simulink model "test_pi_av_formation_event_gazebodirected23a"  (R2023a)
settings: Solver=FixedStepAuto  StartTime=0.0  StopTime=inf  RelTol=1e-3
undefined symbols (not defined in the file or in its folder): angular, DiscIntNeverNeededParam, linear
libraries: ros2lib x28, simulink x8, robotcorelib x8
(part 1 of 4)
settings Model: Creator=johvany  LastModifiedBy=l15
settings OptimizationCC: EnhancedBackFolding=on  PassReuseOutputArgsThreshold=0  ZeroExternalMemoryAtStartup=off  ZeroInternalMemoryAtStartup=off  MaxStackSize=64  OptimizeBlockOrder=speed  DifferentSizesBufferReuse=on  OptimizationCustomize=off
settings DebuggingCC: ParameterTunabilityLossMsg=error
settings HardwareCC: ProdBitPerLong=64  ProdHWDeviceType=Intel->x86-64 (Linux 64)  UseEmbeddedCoderFeatures=off
settings SFSimCC: MATLABDynamicMemAlloc=off
settings RTWCC: Description=Embedded Coder  SystemTargetFile=ert.tlc  HardwareBoard=Robot Operating System 2 (ROS 2)  TLCOptions="-aInlineSetEventsForThisBaseRateFcn=TLC_FALSE -aSuppressMultiTaskScheduler=TLC_FALSE  -aRateBasedStepFcn=0"  TemplateMakefile=ert_default_tmf  Toolchain=Colcon Tools  TargetLang=C++
settings CodeAppCC: ForceParamTrailComments=on  OperatorAnnotations=on
settings ERTTargetCC: ERTCustomFileBanners=off  CodeInterfacePackaging=C++ class  SupportContinuousTime=on  SupportNonInlinedSFcns=on  RemoveResetFunc=off  ModelStepFunctionPrototypeControlCompliant=off  RootIOFormat=Structure reference

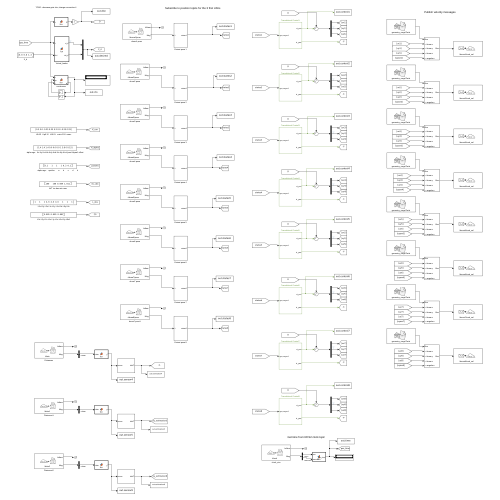
[thumbnail: Simulink's stored preview of the top-level diagram]
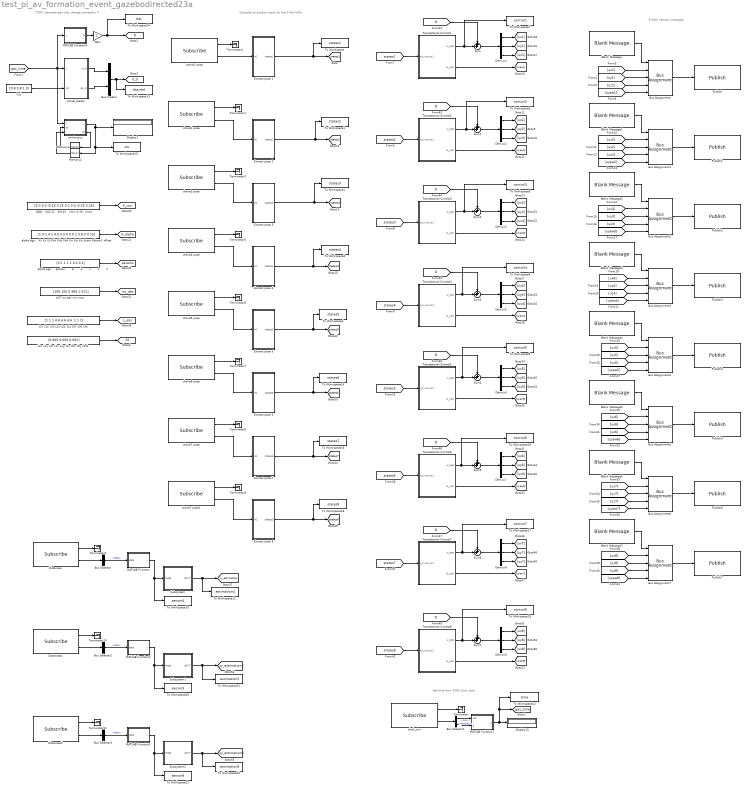
== system test_pi_av_formation_event_gazebodirected23a ==
  note: TODO: decrease gain obs, change connection 4
  note: Publish velocity messages
  note: Subscribe to position topics for the 3 first UAVs
  note: Get time from ROS2 clock topic
  AVT inc dec min max : Constant  Value=[100 100 0.989 1.011]
  Blank Message{,1..7} (8 alike) : ros2lib/Blank Message  messageClass=Message  entityType=geometry_msgs/Twist  messageType=geometry_msgs/Twist  SampleTime=inf
  Bus Assignment{,1..7} (8 alike) : BusAssignment  AssignedSignals=linear.x,linear.y,linear.z,angular.z
  Bus Creator : BusCreator  Inputs=2
  Bus Selector : BusSelector  OutputSignals=data
  Bus Selector1 : BusSelector  OutputSignals=clock.sec,clock.nanosec
  Bus Selector2 : BusSelector  OutputSignals=data
  Bus Selector3 : BusSelector  OutputSignals=data
  Demux{2..9} (8 alike) : Demux  Outputs=3
  Display1 : Display
      settings: Decimation=4
  Display13 : Display
      settings: Decimation=4
  Distances : ros2lib/Subscribe  topicSource=Select from ROS network  topic=/dists  messageType=std_msgs/Float32MultiArray  sampleTime=-1  QOSHistory=Keep last  QOSDepth=1  QOSReliability=Reliable  QOSDurability=Volatile
  Distances1 : ros2lib/Subscribe  topicSource=Select from ROS network  topic=/dists1  messageType=std_msgs/Float32MultiArray  sampleTime=-1  QOSHistory=Keep last  QOSDepth=1  QOSReliability=Reliable  QOSDurability=Volatile
  Distances2 : ros2lib/Subscribe  topicSource=Select from ROS network  topic=/dists2  messageType=std_msgs/Float32MultiArray  sampleTime=-1  QOSHistory=Keep last  QOSDepth=1  QOSReliability=Reliable  QOSDurability=Volatile
  Extract pose 1 : Subsystem
  Extract pose 2 : Subsystem
  Extract pose 3 : Subsystem
  Extract pose 4 : Subsystem
  Extract pose 5 : Subsystem
  Extract pose 6 : Subsystem
  Extract pose 7 : Subsystem
  Extract pose 8 : Subsystem
  Gain : Gain
  L2x L2y L2z L1x L1y L1z L0x L0y L0z : Constant  Value="[1 1 1 4.6 4.6 4.6  1 1 1]"
  L2x L2y L2z L1x L1y L1z L0x L0y L0z1 : Constant  Value=[0.005 0.005 0.002]
  LEAD   Kp0.12   Ki0.01   xmin 0.26  xmax : Constant  Value=[0.3 0.0 -0.25 0.25 0.2 0.0 -0.25 0.25]
  MATLAB Function : MATLAB Function  TreatAsAtomicUnit=on
  MATLAB Function1 : MATLAB Function  TreatAsAtomicUnit=on
  MATLAB Function2 : MATLAB Function  TreatAsAtomicUnit=on
  MATLAB Function3 : MATLAB Function  TreatAsAtomicUnit=on
  MATLAB Function4 : MATLAB Function  TreatAsAtomicUnit=on
  Memory1 : Memory
  Memory2 : Memory
  Publish : ros2lib/Publish  topicSource=Select from ROS network  topic=/drone1/cmd_vel  messageType=geometry_msgs/Twist  QOSHistory=Keep last  QOSDepth=1  QOSReliability=Reliable  QOSDurability=Volatile
  Publish1 : ros2lib/Publish  topicSource=Select from ROS network  topic=/drone2/cmd_vel  messageType=geometry_msgs/Twist  QOSHistory=Keep last  QOSDepth=1  QOSReliability=Reliable  QOSDurability=Volatile
  Publish2 : ros2lib/Publish  topicSource=Select from ROS network  topic=/drone3/cmd_vel  messageType=geometry_msgs/Twist  QOSHistory=Keep last  QOSDepth=1  QOSReliability=Reliable  QOSDurability=Volatile
  Publish3 : ros2lib/Publish  topicSource=Select from ROS network  topic=/drone4/cmd_vel  messageType=geometry_msgs/Twist  QOSHistory=Keep last  QOSDepth=1  QOSReliability=Reliable  QOSDurability=Volatile
  Publish4 : ros2lib/Publish  topicSource=Select from ROS network  topic=/drone5/cmd_vel  messageType=geometry_msgs/Twist  QOSHistory=Keep last  QOSDepth=1  QOSReliability=Reliable  QOSDurability=Volatile
  Publish5 : ros2lib/Publish  topicSource=Select from ROS network  topic=/drone6/cmd_vel  messageType=geometry_msgs/Twist  QOSHistory=Keep last  QOSDepth=1  QOSReliability=Reliable  QOSDurability=Volatile
  Publish6 : ros2lib/Publish  topicSource=Select from ROS network  topic=/drone7/cmd_vel  messageType=geometry_msgs/Twist  QOSHistory=Keep last  QOSDepth=1  QOSReliability=Reliable  QOSDurability=Volatile
  Publish7 : ros2lib/Publish  topicSource=Select from ROS network  topic=/drone8/cmd_vel  messageType=geometry_msgs/Twist  QOSHistory=Keep last  QOSDepth=1  QOSReliability=Reliable  QOSDurability=Volatile
  Subsystem : Subsystem
  Subsystem1 : Subsystem
  Subsystem2 : Subsystem
  Sum{,1..7} (8 alike) : Sum  Inputs=++|
  Terminator{,1..11} (12 alike) : Terminator
  To Workspace : ToWorkspace  VariableName=states1  SampleTime=-1
  To Workspace1 : ToWorkspace  VariableName=states2  SampleTime=-1
  To Workspace10 : ToWorkspace  VariableName=sensor4  SampleTime=-1
  To Workspace11 : ToWorkspace  VariableName=estimation4  SampleTime=-1
  To Workspace12 : ToWorkspace  VariableName=time  SampleTime=-1
  To Workspace13 : ToWorkspace  VariableName=desired  SampleTime=-1
  To Workspace14 : ToWorkspace  VariableName=states6  SampleTime=-1
  To Workspace15 : ToWorkspace  VariableName=control6  SampleTime=-1
  To Workspace16 : ToWorkspace  VariableName=states7  SampleTime=-1
  To Workspace17 : ToWorkspace  VariableName=control7  SampleTime=-1
  To Workspace18 : ToWorkspace  VariableName=states8  SampleTime=-1
  To Workspace19 : ToWorkspace  VariableName=control8  SampleTime=-1
  To Workspace2 : ToWorkspace  VariableName=states3  SampleTime=-1
  To Workspace20 : ToWorkspace  VariableName=sensor5  SampleTime=-1
  To Workspace21 : ToWorkspace  VariableName=estimation5  SampleTime=-1
  To Workspace22 : ToWorkspace  VariableName=sensor8  SampleTime=-1
  To Workspace23 : ToWorkspace  VariableName=estimation8  SampleTime=-1
  To Workspace24 : ToWorkspace  VariableName=dist  SampleTime=-1
  To Workspace25 : ToWorkspace  VariableName=cts  SampleTime=-1
  To Workspace3 : ToWorkspace  VariableName=states4  SampleTime=-1
  To Workspace4 : ToWorkspace  VariableName=states5  SampleTime=-1
  To Workspace5 : ToWorkspace  VariableName=control2  SampleTime=-1
  To Workspace6 : ToWorkspace  VariableName=control3  SampleTime=-1
  To Workspace7 : ToWorkspace  VariableName=control1  SampleTime=-1
  To Workspace8 : ToWorkspace  VariableName=control4  SampleTime=-1
  To Workspace9 : ToWorkspace  VariableName=control5  SampleTime=-1
  Translational Control1 : Subsystem
  Translational Control2 : Subsystem
  Translational Control3 : Subsystem
  Translational Control4 : Subsystem
  Translational Control5 : Subsystem
  Translational Control6 : Subsystem
  Translational Control7 : Subsystem
  Translational Control8 : Subsystem
  Virtual_leader : MATLAB Function  TreatAsAtomicUnit=on
  X_d : Constant  Value=[0.8 0.8 1.3]
  alpha ags:    epsilon       a       b       c       d       h : Constant  Value=[0.1 1 1 1 0.2 0.1]
  alpha ags:   Kx Ky Kz Kdx Kdy Kdz Kix Kiy Kiz Kyaw Kdyaw1 offset : Constant  Value=[1.4 1.4 1.4 0.0 0.0 0.0 1 3.8 0 0.15]
  clock_sim : ros2lib/Subscribe  topicSource=Select from ROS network  topic=/clock  messageType=rosgraph_msgs/Clock  sampleTime=-1  QOSHistory=Keep last  QOSDepth=1  QOSReliability=Reliable  QOSDurability=Volatile
  continuous : MATLAB Function  TreatAsAtomicUnit=on
  drone1 pose : ros2lib/Subscribe  topicSource=Select from ROS network  topic=/drone1/pose  messageType=geometry_msgs/PoseStamped  sampleTime=-1  QOSHistory=Keep last  QOSDepth=1  QOSReliability=Reliable  QOSDurability=Volatile
  drone2 pose : ros2lib/Subscribe  topicSource=Select from ROS network  topic=/drone2/pose  messageType=geometry_msgs/PoseStamped  sampleTime=-1  QOSHistory=Keep last  QOSDepth=1  QOSReliability=Reliable  QOSDurability=Volatile
  drone3 pose : ros2lib/Subscribe  topicSource=Select from ROS network  topic=/drone3/pose  messageType=geometry_msgs/PoseStamped  sampleTime=-1  QOSHistory=Keep last  QOSDepth=1  QOSReliability=Reliable  QOSDurability=Volatile
  drone4 pose : ros2lib/Subscribe  topicSource=Select from ROS network  topic=/drone4/pose  messageType=geometry_msgs/PoseStamped  sampleTime=-1  QOSHistory=Keep last  QOSDepth=1  QOSReliability=Reliable  QOSDurability=Volatile
  drone5 pose : ros2lib/Subscribe  topicSource=Select from ROS network  topic=/drone5/pose  messageType=geometry_msgs/PoseStamped  sampleTime=-1  QOSHistory=Keep last  QOSDepth=1  QOSReliability=Reliable  QOSDurability=Volatile
  drone6 pose : ros2lib/Subscribe  topicSource=Select from ROS network  topic=/drone6/pose  messageType=geometry_msgs/PoseStamped  sampleTime=-1  QOSHistory=Keep last  QOSDepth=1  QOSReliability=Reliable  QOSDurability=Volatile
  drone7 pose : ros2lib/Subscribe  topicSource=Select from ROS network  topic=/drone7/pose  messageType=geometry_msgs/PoseStamped  sampleTime=-1  QOSHistory=Keep last  QOSDepth=1  QOSReliability=Reliable  QOSDurability=Volatile
  drone7 pose1 : ros2lib/Subscribe  topicSource=Select from ROS network  topic=/drone8/pose  messageType=geometry_msgs/PoseStamped  sampleTime=-1  QOSHistory=Keep last  QOSDepth=1  QOSReliability=Reliable  QOSDurability=Volatile
  tag scope: C0=global, D=global, K_alpha=global, K_con=global, L_obs=global, X_d=global, gaz_time=global, inc_dec=global, params=global, states1=global, states2=global, states3=global, states4=global, states5=global, states6=global, states7=global, states8=global, xy_estimation4=global, xy_estimation5=global, xy_estimation8=global
  wires:
  clock_sim/1 -> Terminator/1
  drone2 pose/2 -> Extract pose 2/1(In1)
  drone2 pose/1 -> Terminator1/1
  drone3 pose/2 -> Extract pose 3/1(In1)
  drone3 pose/1 -> Terminator2/1
  Blank Message/1 -> Bus Assignment/1
  Bus Assignment/1 -> Publish/1
  Blank Message1/1 -> Bus Assignment1/1
  Bus Assignment1/1 -> Publish1/1
  Blank Message2/1 -> Bus Assignment2/1
  Bus Assignment2/1 -> Publish2/1
  Blank Message3/1 -> Bus Assignment3/1
  Bus Assignment3/1 -> Publish3/1
  Distances/1 -> Terminator3/1
  Distances/2 -> Bus Selector/1
  Bus Selector/1 -> MATLAB Function/1(data)  "<data>"
  MATLAB Function/1(y) -> To Workspace10/1, Subsystem/1(meas)
  clock_sim/2 -> Bus Selector1/1
  Bus Selector1/1 -> MATLAB Function1/1(sec)  "<sec>"
  Bus Selector1/2 -> MATLAB Function1/2(nanosec)  "<nanosec>"
  Virtual_leader/2(dxi_d) -> Bus Creator/2
  Bus Creator/1 -> To Workspace13/1, [X_d]
  Virtual_leader/1(xi_d) -> Bus Creator/1
  drone1 pose/1 -> Terminator4/1
  drone1 pose/2 -> Extract pose 1/1(In1)
  MATLAB Function1/1(gaz_time) -> To Workspace12/1, [gaz_time], Display13/1
  Extract pose 1/1(states1) -> To Workspace/1, [states1]
  [ux1] -> Bus Assignment/2
  [uy1] -> Bus Assignment/3
  [uz1] -> Bus Assignment/4
  [uyaw1] -> Bus Assignment/5
  X_d/1 -> Virtual_leader/2(Xd)
  Extract pose 2/1(states2) -> To Workspace1/1, [states2]
  Extract pose 3/1(states3) -> To Workspace2/1, [states3]
  drone4 pose/2 -> Extract pose 4/1(In1)
  drone4 pose/1 -> Terminator5/1
  Extract pose 4/1(states4) -> To Workspace3/1, [states4]
  [ux2] -> Bus Assignment1/2
  [uy2] -> Bus Assignment1/3
  [uz2] -> Bus Assignment1/4
  [uyaw2] -> Bus Assignment1/5
  [uy3] -> Bus Assignment2/3
  [uyaw3] -> Bus Assignment2/5
  [uz3] -> Bus Assignment2/4
  [ux3] -> Bus Assignment2/2
  [ux4] -> Bus Assignment3/2
  [uy4] -> Bus Assignment3/3
  [uz4] -> Bus Assignment3/4
  [uyaw4] -> Bus Assignment3/5
  Translational Control1/2(ui_yaw) -> [uyaw1]
  Demux4/2 -> [uy1]
  Demux4/3 -> [uz1]
  [states1] -> Translational Control1/1(xyz,vxvyvz1)
  Translational Control1/1(ui_pos) -> Sum/2, To Workspace7/1
  Demux4/1 -> [ux1]
  LEAD   Kp0.12   Ki0.01   xmin 0.26  xmax/1 -> [K_con]
  alpha ags:   Kx Ky Kz Kdx Kdy Kdz Kix Kiy Kiz Kyaw Kdyaw1 offset/1 -> [K_alpha]
  Demux2/1 -> [ux2]
  Translational Control2/1(ui_pos) -> Sum1/2, To Workspace5/1
  [states2] -> Translational Control2/1(xyz,vxvyvz1)
  Demux2/3 -> [uz2]
  Demux2/2 -> [uy2]
  Translational Control2/2(ui_yaw) -> [uyaw2]
  Translational Control3/2(ui_yaw) -> [uyaw3]
  Demux3/2 -> [uy3]
  Demux3/3 -> [uz3]
  [states3] -> Translational Control3/1(xyz,vxvyvz1)
  Translational Control3/1(ui_pos) -> Sum2/2, To Workspace6/1
  Demux3/1 -> [ux3]
  Demux5/1 -> [ux4]
  Translational Control4/1(ui_pos) -> Sum3/2, To Workspace8/1
  [states4] -> Translational Control4/1(xyz,vxvyvz1)
  Demux5/3 -> [uz4]
  Demux5/2 -> [uy4]
  Translational Control4/2(ui_yaw) -> [uyaw4]
  alpha ags:    epsilon       a       b       c       d       h/1 -> [params]
  AVT inc dec min max/1 -> [inc_dec]
  Subsystem/1(dAVT) -> To Workspace11/1, [xy_estimation4]
  Extract pose 5/1(states5) -> To Workspace4/1, [states5]
  drone5 pose/1 -> Terminator6/1
  drone5 pose/2 -> Extract pose 5/1(In1)
  Bus Assignment4/1 -> Publish4/1
  Blank Message4/1 -> Bus Assignment4/1
  Translational Control5/2(ui_yaw) -> [uyaw5]
  Demux6/2 -> [uy5]
  Demux6/3 -> [uz5]
  [states5] -> Translational Control5/1(xyz,vxvyvz1)
  Translational Control5/1(ui_pos) -> Sum4/2, To Workspace9/1
  Demux6/1 -> [ux5]
  [ux5] -> Bus Assignment4/2
  [uy5] -> Bus Assignment4/3
  [uz5] -> Bus Assignment4/4
  [uyaw5] -> Bus Assignment4/5
  L2x L2y L2z L1x L1y L1z L0x L0y L0z/1 -> [L_obs]
  drone6 pose/2 -> Extract pose 6/1(In1)
  drone6 pose/1 -> Terminator7/1
  Extract pose 6/1(states5) -> [states6], To Workspace14/1
  Demux7/1 -> [ux6]
  Translational Control6/1(ui_pos) -> Sum5/2, To Workspace15/1
  [states6] -> Translational Control6/1(xyz,vxvyvz1)
  Demux7/3 -> [uz6]
  Demux7/2 -> [uy6]
  Translational Control6/2(ui_yaw) -> [uyaw6]
  [uyaw6] -> Bus Assignment5/5
  [uz6] -> Bus Assignment5/4
  [uy6] -> Bus Assignment5/3
  [ux6] -> Bus Assignment5/2
  Blank Message5/1 -> Bus Assignment5/1
  Bus Assignment5/1 -> Publish5/1
  Extract pose 7/1(states5) -> To Workspace16/1, [states7]
  drone7 pose/1 -> Terminator8/1
  drone7 pose/2 -> Extract pose 7/1(In1)
  Bus Assignment6/1 -> Publish6/1
  Blank Message6/1 -> Bus Assignment6/1
  [ux7] -> Bus Assignment6/2
  [uy7] -> Bus Assignment6/3
  [uz7] -> Bus Assignment6/4
  [uyaw7] -> Bus Assignment6/5
  Translational Control7/2(ui_yaw) -> [uyaw7]
  Demux8/2 -> [uy7]
  Demux8/3 -> [uz7]
  [states7] -> Translational Control7/1(xyz,vxvyvz1)
  Translational Control7/1(ui_pos) -> Sum6/2, To Workspace17/1
  Demux8/1 -> [ux7]
  drone7 pose1/2 -> Extract pose 8/1(In1)
  drone7 pose1/1 -> Terminator9/1
  Extract pose 8/1(states5) -> [states8], To Workspace18/1
  [uyaw8] -> Bus Assignment7/5
  [uz8] -> Bus Assignment7/4
  [uy8] -> Bus Assignment7/3
  [ux8] -> Bus Assignment7/2
  Blank Message7/1 -> Bus Assignment7/1
  Bus Assignment7/1 -> Publish7/1
  Demux9/1 -> [ux8]
  Translational Control8/1(ui_pos) -> Sum7/2, To Workspace19/1
  [states8] -> Translational Control8/1(xyz,vxvyvz1)
  Demux9/3 -> [uz8]
  Demux9/2 -> [uy8]
  Translational Control8/2(ui_yaw) -> [uyaw8]
  Subsystem1/1(dAVT) -> To Workspace21/1, [xy_estimation5]
  MATLAB Function2/1(y) -> Subsystem1/1(meas), To Workspace20/1
  Bus Selector2/1 -> MATLAB Function2/1(data)  "<data>"
  Distances1/2 -> Bus Selector2/1
  Distances1/1 -> Terminator10/1
  Distances2/1 -> Terminator11/1
  Distances2/2 -> Bus Selector3/1
  Bus Selector3/1 -> MATLAB Function3/1(data)  "<data>"
  MATLAB Function3/1(y) -> To Workspace22/1, Subsystem2/1(meas)
  Subsystem2/1(dAVT) -> To Workspace23/1, [xy_estimation8]
  MATLAB Function4/1(D) -> Gain/1
  Sum/1 -> Demux4/1
  [D] -> Sum/1
  Sum1/1 -> Demux2/1
  [D] -> Sum1/1
  Sum2/1 -> Demux3/1
  [D] -> Sum2/1
  Sum3/1 -> Demux5/1
  [D] -> Sum3/1
  Sum4/1 -> Demux6/1
  [D] -> Sum4/1
  Sum5/1 -> Demux7/1
  [D] -> Sum6/1
  [D] -> Sum5/1
  Sum6/1 -> Demux8/1
  Sum7/1 -> Demux9/1
  [D] -> Sum7/1
  Gain/1 -> [D], To Workspace24/1
  L2x L2y L2z L1x L1y L1z L0x L0y L0z1/1 -> [C0]
  continuous/1(i) -> Display1/1, To Workspace25/1, Memory2/1
  Memory1/1 -> continuous/2("tp ")
  Memory2/1 -> continuous/3("i ")
  [gaz_time] -> continuous/1(t), MATLAB Function4/1(t), Virtual_leader/1(t)
  continuous/2(tp) -> Memory1/1

== system test_pi_av_formation_event_gazebodirected23a/Extract pose 1 ==
  In1 : Inport
  Bus Creator : BusCreator  Inputs=2
  Bus Selector : BusSelector  OutputSignals=pose.position.x,pose.position.y,pose.position.z,pose.orientation.w,pose.orientation.x,pose.orientation.y,pose.orientation.z
  Demux : Demux  Outputs=3
  Derivative : Derivative
  Discrete Derivative4 : simulink/Discrete/Discrete Derivative  gainval=1.0  ICPrevScaledInput=0.0  OutMin=[]  OutMax=[]  OutDataType=fixdt(1, 16)  OutScaling=2^-10  DoSatur=off
  Mux : Mux  Inputs=3
  Mux1 : Mux  Inputs=2
  Quat to Euler converter : robotcorelib/Coordinate Transformation Conversion  InputRepresentation=Quaternion  InputEulerSequence=ZYX  ShowTrVecInputPort=on  OutputRepresentation=Euler Angles  OutputEulerSequence=XYZ  ShowTrVecOutputPort=on  SimulateUsing=Interpreted execution
      settings: LibrarySourceBlock=roslib/Utilities/Coordinate Transformation Conversion
  Vector Concatenate : Concatenate  NumInputs=4
  states1 : Outport
  wires:
  Bus Selector/5 -> Vector Concatenate/2  "<x>"
  Quat to Euler converter/1 -> Demux/1
  Bus Selector/6 -> Vector Concatenate/3  "<y>"
  Bus Selector/1 -> Mux/1  "<x>"
  Bus Selector/7 -> Vector Concatenate/4  "<z>"
  Vector Concatenate/1 -> Quat to Euler converter/1
  In1/1 -> Bus Selector/1
  Bus Selector/4 -> Vector Concatenate/1  "<w>"
  Bus Selector/2 -> Mux/2  "<y>"
  Bus Selector/3 -> Mux/3  "<z>"
  Demux/3 -> Derivative/1, Mux1/1  "yaw"
  Mux/1 -> Bus Creator/1  "xyz"
  Bus Creator/1 -> states1/1
  Derivative/1 -> Mux1/2
  Mux1/1 -> Bus Creator/2  "YAW"

== system test_pi_av_formation_event_gazebodirected23a/Extract pose 2 ==
  In1 : Inport
  Bus Creator : BusCreator  Inputs=2
  Bus Selector : BusSelector  OutputSignals=pose.position.x,pose.position.y,pose.position.z,pose.orientation.w,pose.orientation.x,pose.orientation.y,pose.orientation.z
  Demux : Demux  Outputs=3
  Derivative : Derivative
  Discrete Derivative4 : simulink/Discrete/Discrete Derivative  gainval=1.0  ICPrevScaledInput=0.0  OutMin=[]  OutMax=[]  OutDataType=fixdt(1, 16)  OutScaling=2^-10  DoSatur=off
  Mux : Mux  Inputs=3
  Mux1 : Mux  Inputs=2
  Quat to Euler converter : robotcorelib/Coordinate Transformation Conversion  InputRepresentation=Quaternion  InputEulerSequence=ZYX  ShowTrVecInputPort=on  OutputRepresentation=Euler Angles  OutputEulerSequence=XYZ  ShowTrVecOutputPort=on  SimulateUsing=Interpreted execution
      settings: LibrarySourceBlock=roslib/Utilities/Coordinate Transformation Conversion
  Vector Concatenate : Concatenate  NumInputs=4
  states2 : Outport
  wires:
  Mux1/1 -> Bus Creator/2  "YAW"
  Derivative/1 -> Mux1/2
  Bus Creator/1 -> states2/1
  Mux/1 -> Bus Creator/1  "xyz"
  Demux/3 -> Mux1/1, Derivative/1  "yaw"
  Bus Selector/3 -> Mux/3  "<z>"
  Bus Selector/2 -> Mux/2  "<y>"
  Bus Selector/4 -> Vector Concatenate/1  "<w>"
  In1/1 -> Bus Selector/1
  Vector Concatenate/1 -> Quat to Euler converter/1
  Bus Selector/7 -> Vector Concatenate/4  "<z>"
  Bus Selector/1 -> Mux/1  "<x>"
  Bus Selector/6 -> Vector Concatenate/3  "<y>"
  Quat to Euler converter/1 -> Demux/1
  Bus Selector/5 -> Vector Concatenate/2  "<x>"

== system test_pi_av_formation_event_gazebodirected23a/Extract pose 3 ==
  In1 : Inport
  Bus Creator : BusCreator  Inputs=2
  Bus Selector : BusSelector  OutputSignals=pose.position.x,pose.position.y,pose.position.z,pose.orientation.w,pose.orientation.x,pose.orientation.y,pose.orientation.z
  Demux : Demux  Outputs=3
  Derivative : Derivative
  Discrete Derivative4 : simulink/Discrete/Discrete Derivative  gainval=1.0  ICPrevScaledInput=0.0  OutMin=[]  OutMax=[]  OutDataType=fixdt(1, 16)  OutScaling=2^-10  DoSatur=off
  Mux : Mux  Inputs=3
  Mux1 : Mux  Inputs=2
  Quat to Euler converter : robotcorelib/Coordinate Transformation Conversion  InputRepresentation=Quaternion  InputEulerSequence=ZYX  ShowTrVecInputPort=on  OutputRepresentation=Euler Angles  OutputEulerSequence=XYZ  ShowTrVecOutputPort=on  SimulateUsing=Interpreted execution
      settings: LibrarySourceBlock=roslib/Utilities/Coordinate Transformation Conversion
  Vector Concatenate : Concatenate  NumInputs=4
  states3 : Outport
  wires:
  Bus Selector/5 -> Vector Concatenate/2  "<x>"
  Quat to Euler converter/1 -> Demux/1
  Bus Selector/6 -> Vector Concatenate/3  "<y>"
  Bus Selector/1 -> Mux/1  "<x>"
  Bus Selector/7 -> Vector Concatenate/4  "<z>"
  Vector Concatenate/1 -> Quat to Euler converter/1
  In1/1 -> Bus Selector/1
  Bus Selector/4 -> Vector Concatenate/1  "<w>"
  Bus Selector/2 -> Mux/2  "<y>"
  Bus Selector/3 -> Mux/3  "<z>"
  Demux/3 -> Derivative/1, Mux1/1  "yaw"
  Mux/1 -> Bus Creator/1  "xyz"
  Bus Creator/1 -> states3/1
  Derivative/1 -> Mux1/2
  Mux1/1 -> Bus Creator/2  "YAW"

== system test_pi_av_formation_event_gazebodirected23a/Extract pose 4 ==
  In1 : Inport
  Bus Creator : BusCreator  Inputs=2
  Bus Selector : BusSelector  OutputSignals=pose.position.x,pose.position.y,pose.position.z,pose.orientation.w,pose.orientation.x,pose.orientation.y,pose.orientation.z
  Demux : Demux  Outputs=3
  Derivative : Derivative
  Discrete Derivative4 : simulink/Discrete/Discrete Derivative  gainval=1.0  ICPrevScaledInput=0.0  OutMin=[]  OutMax=[]  OutDataType=fixdt(1, 16)  OutScaling=2^-10  DoSatur=off
  Mux : Mux  Inputs=3
  Mux1 : Mux  Inputs=2
  Quat to Euler converter : robotcorelib/Coordinate Transformation Conversion  InputRepresentation=Quaternion  InputEulerSequence=ZYX  ShowTrVecInputPort=on  OutputRepresentation=Euler Angles  OutputEulerSequence=XYZ  ShowTrVecOutputPort=on  SimulateUsing=Interpreted execution
      settings: LibrarySourceBlock=roslib/Utilities/Coordinate Transformation Conversion
  Vector Concatenate : Concatenate  NumInputs=4
  states4 : Outport
  wires:
  Mux1/1 -> Bus Creator/2  "YAW"
  Derivative/1 -> Mux1/2
  Bus Creator/1 -> states4/1
  Mux/1 -> Bus Creator/1  "xyz"
  Demux/3 -> Mux1/1, Derivative/1  "yaw"
  Bus Selector/3 -> Mux/3  "<z>"
  Bus Selector/2 -> Mux/2  "<y>"
  Bus Selector/4 -> Vector Concatenate/1  "<w>"
  In1/1 -> Bus Selector/1
  Vector Concatenate/1 -> Quat to Euler converter/1
  Bus Selector/7 -> Vector Concatenate/4  "<z>"
  Bus Selector/1 -> Mux/1  "<x>"
  Bus Selector/6 -> Vector Concatenate/3  "<y>"
  Quat to Euler converter/1 -> Demux/1
  Bus Selector/5 -> Vector Concatenate/2  "<x>"

== system test_pi_av_formation_event_gazebodirected23a/Extract pose 5 ==
  In1 : Inport
  Bus Creator : BusCreator  Inputs=2
  Bus Selector : BusSelector  OutputSignals=pose.position.x,pose.position.y,pose.position.z,pose.orientation.w,pose.orientation.x,pose.orientation.y,pose.orientation.z
  Demux : Demux  Outputs=3
  Derivative : Derivative
  Discrete Derivative4 : simulink/Discrete/Discrete Derivative  gainval=1.0  ICPrevScaledInput=0.0  OutMin=[]  OutMax=[]  OutDataType=fixdt(1, 16)  OutScaling=2^-10  DoSatur=off
  Mux : Mux  Inputs=3
  Mux1 : Mux  Inputs=2
  Quat to Euler converter : robotcorelib/Coordinate Transformation Conversion  InputRepresentation=Quaternion  InputEulerSequence=ZYX  ShowTrVecInputPort=on  OutputRepresentation=Euler Angles  OutputEulerSequence=XYZ  ShowTrVecOutputPort=on  SimulateUsing=Interpreted execution
      settings: LibrarySourceBlock=roslib/Utilities/Coordinate Transformation Conversion
  Vector Concatenate : Concatenate  NumInputs=4
  states5 : Outport
  wires:
  Bus Selector/5 -> Vector Concatenate/2  "<x>"
  Quat to Euler converter/1 -> Demux/1
  Bus Selector/6 -> Vector Concatenate/3  "<y>"
  Bus Selector/1 -> Mux/1  "<x>"
  Bus Selector/7 -> Vector Concatenate/4  "<z>"
  Vector Concatenate/1 -> Quat to Euler converter/1
  In1/1 -> Bus Selector/1
  Bus Selector/4 -> Vector Concatenate/1  "<w>"
  Bus Selector/2 -> Mux/2  "<y>"
  Bus Selector/3 -> Mux/3  "<z>"
  Demux/3 -> Derivative/1, Mux1/1  "yaw"
  Mux/1 -> Bus Creator/1  "xyz"
  Bus Creator/1 -> states5/1
  Derivative/1 -> Mux1/2
  Mux1/1 -> Bus Creator/2  "YAW"

== system test_pi_av_formation_event_gazebodirected23a/Extract pose 6 ==
  In1 : Inport
  Bus Creator : BusCreator  Inputs=2
  Bus Selector : BusSelector  OutputSignals=pose.position.x,pose.position.y,pose.position.z,pose.orientation.w,pose.orientation.x,pose.orientation.y,pose.orientation.z
  Demux : Demux  Outputs=3
  Derivative : Derivative
  Discrete Derivative4 : simulink/Discrete/Discrete Derivative  gainval=1.0  ICPrevScaledInput=0.0  OutMin=[]  OutMax=[]  OutDataType=fixdt(1, 16)  OutScaling=2^-10  DoSatur=off
  Mux : Mux  Inputs=3
  Mux1 : Mux  Inputs=2
  Quat to Euler converter : robotcorelib/Coordinate Transformation Conversion  InputRepresentation=Quaternion  InputEulerSequence=ZYX  ShowTrVecInputPort=on  OutputRepresentation=Euler Angles  OutputEulerSequence=XYZ  ShowTrVecOutputPort=on  SimulateUsing=Interpreted execution
      settings: LibrarySourceBlock=roslib/Utilities/Coordinate Transformation Conversion
  Vector Concatenate : Concatenate  NumInputs=4
  states5 : Outport
  wires:
  Mux1/1 -> Bus Creator/2  "YAW"
  Derivative/1 -> Mux1/2
  Bus Creator/1 -> states5/1
  Mux/1 -> Bus Creator/1  "xyz"
  Demux/3 -> Mux1/1, Derivative/1  "yaw"
  Bus Selector/3 -> Mux/3  "<z>"
  Bus Selector/2 -> Mux/2  "<y>"
  Bus Selector/4 -> Vector Concatenate/1  "<w>"
  In1/1 -> Bus Selector/1
  Vector Concatenate/1 -> Quat to Euler converter/1
  Bus Selector/7 -> Vector Concatenate/4  "<z>"
  Bus Selector/1 -> Mux/1  "<x>"
  Bus Selector/6 -> Vector Concatenate/3  "<y>"
  Quat to Euler converter/1 -> Demux/1
  Bus Selector/5 -> Vector Concatenate/2  "<x>"

== system test_pi_av_formation_event_gazebodirected23a/Extract pose 7 ==
  In1 : Inport
  Bus Creator : BusCreator  Inputs=2
  Bus Selector : BusSelector  OutputSignals=pose.position.x,pose.position.y,pose.position.z,pose.orientation.w,pose.orientation.x,pose.orientation.y,pose.orientation.z
  Demux : Demux  Outputs=3
  Derivative : Derivative
  Discrete Derivative4 : simulink/Discrete/Discrete Derivative  gainval=1.0  ICPrevScaledInput=0.0  OutMin=[]  OutMax=[]  OutDataType=fixdt(1, 16)  OutScaling=2^-10  DoSatur=off
  Mux : Mux  Inputs=3
  Mux1 : Mux  Inputs=2
  Quat to Euler converter : robotcorelib/Coordinate Transformation Conversion  InputRepresentation=Quaternion  InputEulerSequence=ZYX  ShowTrVecInputPort=on  OutputRepresentation=Euler Angles  OutputEulerSequence=XYZ  ShowTrVecOutputPort=on  SimulateUsing=Interpreted execution
      settings: LibrarySourceBlock=roslib/Utilities/Coordinate Transformation Conversion
  Vector Concatenate : Concatenate  NumInputs=4
  states5 : Outport
  wires:
  Bus Selector/5 -> Vector Concatenate/2  "<x>"
  Quat to Euler converter/1 -> Demux/1
  Bus Selector/6 -> Vector Concatenate/3  "<y>"
  Bus Selector/1 -> Mux/1  "<x>"
  Bus Selector/7 -> Vector Concatenate/4  "<z>"
  Vector Concatenate/1 -> Quat to Euler converter/1
  In1/1 -> Bus Selector/1
  Bus Selector/4 -> Vector Concatenate/1  "<w>"
  Bus Selector/2 -> Mux/2  "<y>"
  Bus Selector/3 -> Mux/3  "<z>"
  Demux/3 -> Derivative/1, Mux1/1  "yaw"
  Mux/1 -> Bus Creator/1  "xyz"
  Bus Creator/1 -> states5/1
  Derivative/1 -> Mux1/2
  Mux1/1 -> Bus Creator/2  "YAW"

== system test_pi_av_formation_event_gazebodirected23a/Extract pose 8 ==
  In1 : Inport
  Bus Creator : BusCreator  Inputs=2
  Bus Selector : BusSelector  OutputSignals=pose.position.x,pose.position.y,pose.position.z,pose.orientation.w,pose.orientation.x,pose.orientation.y,pose.orientation.z
  Demux : Demux  Outputs=3
  Derivative : Derivative
  Discrete Derivative4 : simulink/Discrete/Discrete Derivative  gainval=1.0  ICPrevScaledInput=0.0  OutMin=[]  OutMax=[]  OutDataType=fixdt(1, 16)  OutScaling=2^-10  DoSatur=off
  Mux : Mux  Inputs=3
  Mux1 : Mux  Inputs=2
  Quat to Euler converter : robotcorelib/Coordinate Transformation Conversion  InputRepresentation=Quaternion  InputEulerSequence=ZYX  ShowTrVecInputPort=on  OutputRepresentation=Euler Angles  OutputEulerSequence=XYZ  ShowTrVecOutputPort=on  SimulateUsing=Interpreted execution
      settings: LibrarySourceBlock=roslib/Utilities/Coordinate Transformation Conversion
  Vector Concatenate : Concatenate  NumInputs=4
  states5 : Outport
  wires:
  Mux1/1 -> Bus Creator/2  "YAW"
  Derivative/1 -> Mux1/2
  Bus Creator/1 -> states5/1
  Mux/1 -> Bus Creator/1  "xyz"
  Demux/3 -> Mux1/1, Derivative/1  "yaw"
  Bus Selector/3 -> Mux/3  "<z>"
  Bus Selector/2 -> Mux/2  "<y>"
  Bus Selector/4 -> Vector Concatenate/1  "<w>"
  In1/1 -> Bus Selector/1
  Vector Concatenate/1 -> Quat to Euler converter/1
  Bus Selector/7 -> Vector Concatenate/4  "<z>"
  Bus Selector/1 -> Mux/1  "<x>"
  Bus Selector/6 -> Vector Concatenate/3  "<y>"
  Quat to Euler converter/1 -> Demux/1
  Bus Selector/5 -> Vector Concatenate/2  "<x>"

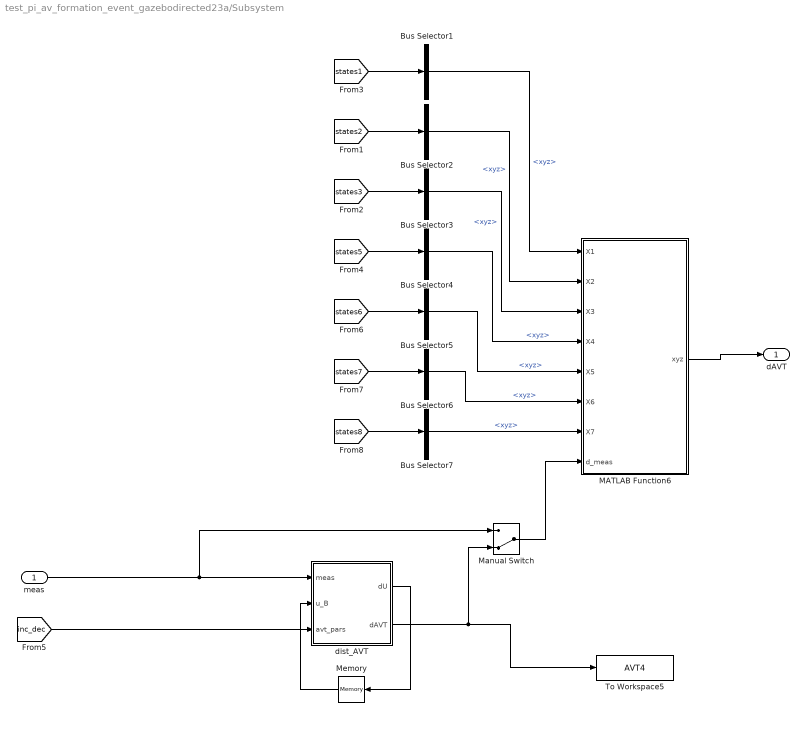
== system test_pi_av_formation_event_gazebodirected23a/Subsystem ==
  meas : Inport
  Bus Selector{1..7} (7 alike) : BusSelector  OutputSignals=xyz
  MATLAB Function6 : MATLAB Function  TreatAsAtomicUnit=on
  Manual Switch : ManualSwitch  CurrentSetting=0
  Memory : Memory  InitialCondition=[1 0.5 0 1 0.5 0 1 0.5 0 1 0.5 0 1 0.5 0 1 0.5 0 1 0.5 0]
  To Workspace5 : ToWorkspace  VariableName=AVT4  SampleTime=-1
  dist_AVT : MATLAB Function  Tag=Outer control  TreatAsAtomicUnit=on
  dAVT : Outport
  wires:
  Memory/1 -> dist_AVT/2(u_B)
  dist_AVT/2(dAVT) -> Manual Switch/2, To Workspace5/1
  dist_AVT/1(dU) -> Memory/1
  meas/1 -> Manual Switch/1, dist_AVT/1(meas)
  [inc_dec] -> dist_AVT/3(avt_pars)
  MATLAB Function6/1(xyz) -> dAVT/1
  [states1] -> Bus Selector1/1
  Bus Selector1/1 -> MATLAB Function6/1(X1)  "<xyz>"
  [states2] -> Bus Selector2/1
  [states3] -> Bus Selector3/1
  Bus Selector2/1 -> MATLAB Function6/2(X2)  "<xyz>"
  Bus Selector3/1 -> MATLAB Function6/3(X3)  "<xyz>"
  [states5] -> Bus Selector4/1
  Bus Selector4/1 -> MATLAB Function6/4(X4)  "<xyz>"
  Manual Switch/1 -> MATLAB Function6/8(d_meas)
  Bus Selector5/1 -> MATLAB Function6/5(X5)  "<xyz>"
  [states6] -> Bus Selector5/1
  [states7] -> Bus Selector6/1
  Bus Selector6/1 -> MATLAB Function6/6(X6)  "<xyz>"
  [states8] -> Bus Selector7/1
  Bus Selector7/1 -> MATLAB Function6/7(X7)  "<xyz>"

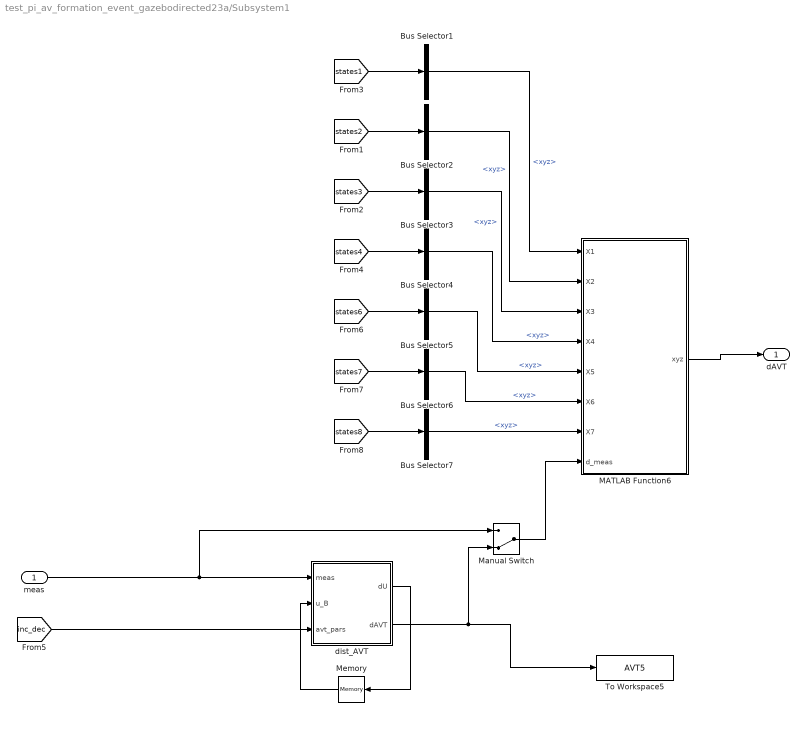
== system test_pi_av_formation_event_gazebodirected23a/Subsystem1 ==
  meas : Inport
  Bus Selector{1..7} (7 alike) : BusSelector  OutputSignals=xyz
  MATLAB Function6 : MATLAB Function  TreatAsAtomicUnit=on
  Manual Switch : ManualSwitch  CurrentSetting=0
  Memory : Memory  InitialCondition=[1 0.5 0 1 0.5 0 1 0.5 0 1 0.5 0 1 0.5 0 1 0.5 0 1 0.5 0]
  To Workspace5 : ToWorkspace  VariableName=AVT5  SampleTime=-1
  dist_AVT : MATLAB Function  Tag=Outer control  TreatAsAtomicUnit=on
  dAVT : Outport
  wires:
  Bus Selector7/1 -> MATLAB Function6/7(X7)  "<xyz>"
  [states8] -> Bus Selector7/1
  Bus Selector6/1 -> MATLAB Function6/6(X6)  "<xyz>"
  [states7] -> Bus Selector6/1
  [states6] -> Bus Selector5/1
  Bus Selector5/1 -> MATLAB Function6/5(X5)  "<xyz>"
  Manual Switch/1 -> MATLAB Function6/8(d_meas)
  Bus Selector4/1 -> MATLAB Function6/4(X4)  "<xyz>"
  [states4] -> Bus Selector4/1
  Bus Selector3/1 -> MATLAB Function6/3(X3)  "<xyz>"
  Bus Selector2/1 -> MATLAB Function6/2(X2)  "<xyz>"
  [states3] -> Bus Selector3/1
  [states2] -> Bus Selector2/1
  Bus Selector1/1 -> MATLAB Function6/1(X1)  "<xyz>"
  [states1] -> Bus Selector1/1
  MATLAB Function6/1(xyz) -> dAVT/1
  [inc_dec] -> dist_AVT/3(avt_pars)
  meas/1 -> dist_AVT/1(meas), Manual Switch/1
  dist_AVT/1(dU) -> Memory/1
  dist_AVT/2(dAVT) -> To Workspace5/1, Manual Switch/2
  Memory/1 -> dist_AVT/2(u_B)

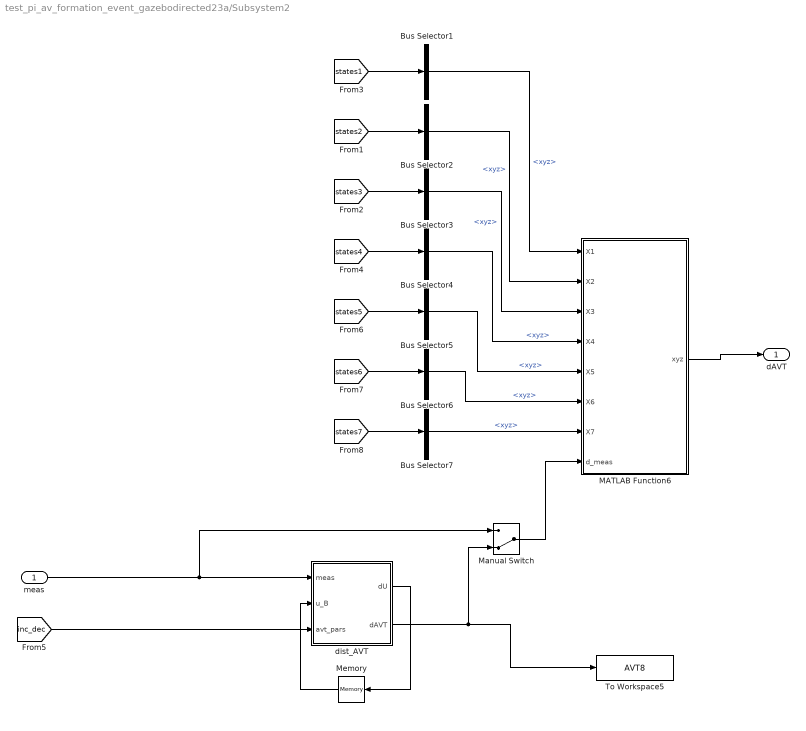
== system test_pi_av_formation_event_gazebodirected23a/Subsystem2 ==
  meas : Inport
  Bus Selector{1..7} (7 alike) : BusSelector  OutputSignals=xyz
  MATLAB Function6 : MATLAB Function  TreatAsAtomicUnit=on
  Manual Switch : ManualSwitch  CurrentSetting=0
  Memory : Memory  InitialCondition=[1 0.5 0 1 0.5 0 1 0.5 0 1 0.5 0 1 0.5 0 1 0.5 0 1 0.5 0]
  To Workspace5 : ToWorkspace  VariableName=AVT8  SampleTime=-1
  dist_AVT : MATLAB Function  Tag=Outer control  TreatAsAtomicUnit=on
  dAVT : Outport
  wires:
  Memory/1 -> dist_AVT/2(u_B)
  dist_AVT/2(dAVT) -> Manual Switch/2, To Workspace5/1
  dist_AVT/1(dU) -> Memory/1
  meas/1 -> Manual Switch/1, dist_AVT/1(meas)
  [inc_dec] -> dist_AVT/3(avt_pars)
  MATLAB Function6/1(xyz) -> dAVT/1
  [states1] -> Bus Selector1/1
  Bus Selector1/1 -> MATLAB Function6/1(X1)  "<xyz>"
  [states2] -> Bus Selector2/1
  [states3] -> Bus Selector3/1
  Bus Selector2/1 -> MATLAB Function6/2(X2)  "<xyz>"
  Bus Selector3/1 -> MATLAB Function6/3(X3)  "<xyz>"
  [states4] -> Bus Selector4/1
  Bus Selector4/1 -> MATLAB Function6/4(X4)  "<xyz>"
  Manual Switch/1 -> MATLAB Function6/8(d_meas)
  Bus Selector5/1 -> MATLAB Function6/5(X5)  "<xyz>"
  [states5] -> Bus Selector5/1
  [states6] -> Bus Selector6/1
  Bus Selector6/1 -> MATLAB Function6/6(X6)  "<xyz>"
  [states7] -> Bus Selector7/1
  Bus Selector7/1 -> MATLAB Function6/7(X7)  "<xyz>"

== system test_pi_av_formation_event_gazebodirected23a/Translational Control1 ==
  xyz,vxvyvz1 : Inport
  Flocking1 : Subsystem
  ui_pos : Outport  VectorParamsAs1DForOutWhenUnconnected=off
  ui_yaw : Outport  Port=2  VectorParamsAs1DForOutWhenUnconnected=off
  wires:
  xyz,vxvyvz1/1 -> Flocking1/4(state)
  [states2] -> Flocking1/5(statej)
  [states3] -> Flocking1/3(ref2), Flocking1/6(statek)
  [states4] -> Flocking1/7(statel)
  Flocking1/1(U_ipos) -> ui_pos/1
  Flocking1/2(U_iyaw) -> ui_yaw/1
  [states5] -> Flocking1/8(statem)
  [states6] -> Flocking1/9(staten)
  [states7] -> Flocking1/10(stateo)
  [states8] -> Flocking1/2(ref1), Flocking1/11(statep)
  [X_d] -> Flocking1/1(ref)

== system test_pi_av_formation_event_gazebodirected23a/Translational Control2 ==
  xyz,vxvyvz1 : Inport
  Flocking1 : Subsystem
  ui_pos : Outport  VectorParamsAs1DForOutWhenUnconnected=off
  ui_yaw : Outport  Port=2  VectorParamsAs1DForOutWhenUnconnected=off
  wires:
  Flocking1/2(U_iyaw) -> ui_yaw/1
  Flocking1/1(U_ipos) -> ui_pos/1
  [states4] -> Flocking1/6(statel)
  [states3] -> Flocking1/5(statek)
  [states1] -> Flocking1/4(statej)
  xyz,vxvyvz1/1 -> Flocking1/3(state)
  [states5] -> Flocking1/2(ref1), Flocking1/7(statem)
  [states6] -> Flocking1/8(staten)
  [states7] -> Flocking1/9(stateo)
  [states8] -> Flocking1/10(statep)
  [X_d] -> Flocking1/1(ref)

== system test_pi_av_formation_event_gazebodirected23a/Translational Control3 ==
  xyz,vxvyvz1 : Inport
  Flocking1 : Subsystem
  ui_pos : Outport  VectorParamsAs1DForOutWhenUnconnected=off
  ui_yaw : Outport  Port=2  VectorParamsAs1DForOutWhenUnconnected=off
  wires:
  xyz,vxvyvz1/1 -> Flocking1/3(state)
  [states1] -> Flocking1/4(statej)
  [states2] -> Flocking1/5(statek)
  [states4] -> Flocking1/6(statel)
  Flocking1/1(U_ipos) -> ui_pos/1
  Flocking1/2(U_iyaw) -> ui_yaw/1
  [states5] -> Flocking1/7(statem)
  [X_d] -> Flocking1/1(ref)
  [states6] -> Flocking1/8(staten)
  [states7] -> Flocking1/2(ref1), Flocking1/9(stateo)
  [states8] -> Flocking1/10(stateo1)

== system test_pi_av_formation_event_gazebodirected23a/Translational Control4 ==
  xyz,vxvyvz1 : Inport
  Flocking1 : Subsystem
  ui_pos : Outport  VectorParamsAs1DForOutWhenUnconnected=off
  ui_yaw : Outport  Port=2  VectorParamsAs1DForOutWhenUnconnected=off
  wires:
  Flocking1/2(U_iyaw) -> ui_yaw/1
  Flocking1/1(U_ipos) -> ui_pos/1
  [states3] -> Flocking1/7(statel)
  [states2] -> Flocking1/2(ref1), Flocking1/6(statek)
  [states1] -> Flocking1/5(statej)
  xyz,vxvyvz1/1 -> Flocking1/4(state)
  [states5] -> Flocking1/8(statem)
  [states6] -> Flocking1/9(statem1)
  [states7] -> Flocking1/3(ref2), Flocking1/10(stateo)
  [states8] -> Flocking1/11(stateo1)
  [X_d] -> Flocking1/1(ref)

== system test_pi_av_formation_event_gazebodirected23a/Translational Control5 ==
  xyz,vxvyvz1 : Inport
  Flocking1 : Subsystem
  ui_pos : Outport  VectorParamsAs1DForOutWhenUnconnected=off
  ui_yaw : Outport  Port=2  VectorParamsAs1DForOutWhenUnconnected=off
  wires:
  [states4] -> Flocking1/7(statem)
  xyz,vxvyvz1/1 -> Flocking1/3(state)
  [states1] -> Flocking1/4(statej)
  [states2] -> Flocking1/5(statek)
  [states3] -> Flocking1/2(ref1), Flocking1/6(statel)
  Flocking1/1(U_ipos) -> ui_pos/1
  Flocking1/2(U_iyaw) -> ui_yaw/1
  [states6] -> Flocking1/8(staten)
  [states7] -> Flocking1/9(stateo)
  [states8] -> Flocking1/10(stateo1)
  [X_d] -> Flocking1/1(ref)

== system test_pi_av_formation_event_gazebodirected23a/Translational Control6 ==
  xyz,vxvyvz1 : Inport
  Flocking1 : Subsystem
  ui_pos : Outport  VectorParamsAs1DForOutWhenUnconnected=off
  ui_yaw : Outport  Port=2  VectorParamsAs1DForOutWhenUnconnected=off
  wires:
  Flocking1/2(U_iyaw) -> ui_yaw/1
  Flocking1/1(U_ipos) -> ui_pos/1
  [states3] -> Flocking1/2(ref1), Flocking1/7(statel)
  [states2] -> Flocking1/6(statek)
  [states1] -> Flocking1/5(statej)
  xyz,vxvyvz1/1 -> Flocking1/4(state)
  [states4] -> Flocking1/8(statem)
  [states5] -> Flocking1/3(ref2), Flocking1/9(staten)
  [states7] -> Flocking1/10(staten1)
  [states8] -> Flocking1/11(staten2)
  [X_d] -> Flocking1/1(ref)

== system test_pi_av_formation_event_gazebodirected23a/Translational Control7 ==
  xyz,vxvyvz1 : Inport
  Flocking1 : Subsystem
  ui_pos : Outport  VectorParamsAs1DForOutWhenUnconnected=off
  ui_yaw : Outport  Port=2  VectorParamsAs1DForOutWhenUnconnected=off
  wires:
  [states6] -> Flocking1/10(stateo)
  [states5] -> Flocking1/9(staten)
  [states4] -> Flocking1/8(statem)
  xyz,vxvyvz1/1 -> Flocking1/4(state)
  [states1] -> Flocking1/5(statej)
  [states2] -> Flocking1/3(ref2), Flocking1/6(statek)
  [states3] -> Flocking1/2(ref1), Flocking1/7(statel)
  Flocking1/1(U_ipos) -> ui_pos/1
  Flocking1/2(U_iyaw) -> ui_yaw/1
  [states8] -> Flocking1/11(stateo1)
  [X_d] -> Flocking1/1(ref)

== system test_pi_av_formation_event_gazebodirected23a/Translational Control8 ==
  xyz,vxvyvz1 : Inport
  Flocking1 : Subsystem
  ui_pos : Outport  VectorParamsAs1DForOutWhenUnconnected=off
  ui_yaw : Outport  Port=2  VectorParamsAs1DForOutWhenUnconnected=off
  wires:
  [states7] -> Flocking1/11(stateo1)
  Flocking1/2(U_iyaw) -> ui_yaw/1
  Flocking1/1(U_ipos) -> ui_pos/1
  [states3] -> Flocking1/3(ref2), Flocking1/7(statel)
  [states2] -> Flocking1/6(statek)
  [states1] -> Flocking1/2(ref1), Flocking1/5(statej)
  xyz,vxvyvz1/1 -> Flocking1/4(state)
  [states4] -> Flocking1/8(statem)
  [states5] -> Flocking1/9(staten)
  [states6] -> Flocking1/10(stateo)
  [X_d] -> Flocking1/1(ref)

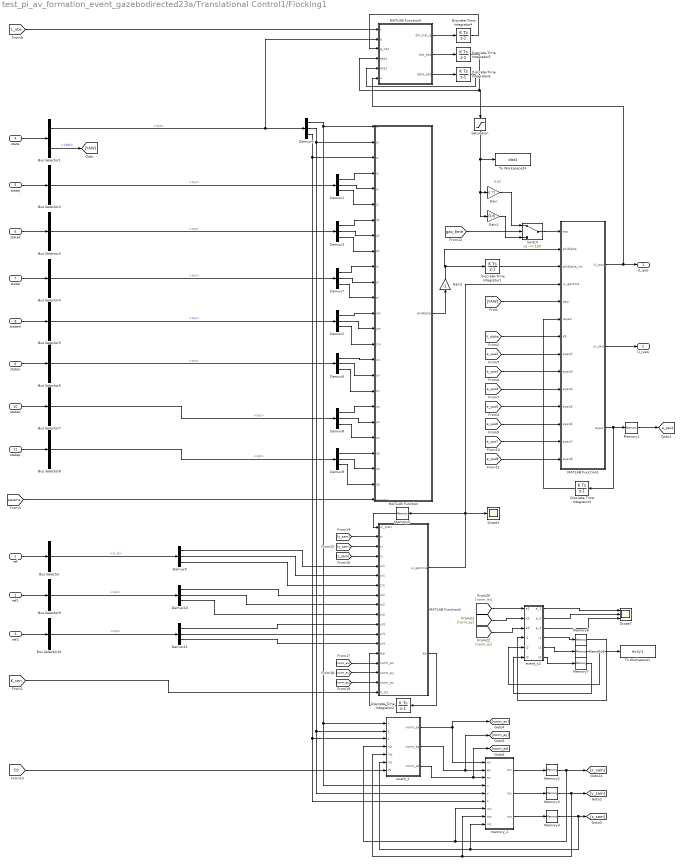
== system test_pi_av_formation_event_gazebodirected23a/Translational Control1/Flocking1 ==
  note: 0.62
  ref : Inport
  ref1 : Inport  Port=2
  ref2 : Inport  Port=3
  state : Inport  Port=4
  statej : Inport  Port=5
  statek : Inport  Port=6
  statel : Inport  Port=7
  statem : Inport  Port=8
  staten : Inport  Port=9
  stateo : Inport  Port=10
  statep : Inport  Port=11
  Bus Selector : BusSelector  OutputSignals=xi_d
  Bus Selector1 : BusSelector  OutputSignals=xyz,YAW
  Bus Selector{2..10} (9 alike) : BusSelector  OutputSignals=xyz
  Demux{1..11} (11 alike) : Demux  Outputs=3
  Discrete-Time Integrator1 : DiscreteIntegrator  SampleTime=-1  LimitOutput=on  UpperSaturationLimit=2  LowerSaturationLimit=-2  ICPrevOutput=DiscIntNeverNeededParam  ICPrevScaledInput=DiscIntNeverNeededParam
  Discrete-Time Integrator2 : DiscreteIntegrator  SampleTime=-1  LimitOutput=on  UpperSaturationLimit=2  LowerSaturationLimit=-2  ICPrevOutput=DiscIntNeverNeededParam  ICPrevScaledInput=DiscIntNeverNeededParam
  Discrete-Time Integrator3 : DiscreteIntegrator  SampleTime=-1  LimitOutput=on  UpperSaturationLimit=1  LowerSaturationLimit=-1  ICPrevOutput=DiscIntNeverNeededParam  ICPrevScaledInput=DiscIntNeverNeededParam
  Discrete-Time Integrator4 : DiscreteIntegrator  SampleTime=-1  LimitOutput=on  UpperSaturationLimit=5  LowerSaturationLimit=-5  ICPrevOutput=DiscIntNeverNeededParam  ICPrevScaledInput=DiscIntNeverNeededParam
  Discrete-Time Integrator5 : DiscreteIntegrator  SampleTime=-1  LimitOutput=on  UpperSaturationLimit=5  LowerSaturationLimit=-5  ICPrevOutput=DiscIntNeverNeededParam  ICPrevScaledInput=DiscIntNeverNeededParam
  Discrete-Time Integrator6 : DiscreteIntegrator  SampleTime=-1  LimitOutput=on  UpperSaturationLimit=0.2  LowerSaturationLimit=-0.2  ICPrevOutput=DiscIntNeverNeededParam  ICPrevScaledInput=DiscIntNeverNeededParam
  Gain : Gain  Gain=0.77
  Gain1 : Gain  Gain=0.6
  Gain2 : Gain  Gain=-1
  MATLAB Function : MATLAB Function  TreatAsAtomicUnit=on
  MATLAB Function1 : MATLAB Function  TreatAsAtomicUnit=on
  MATLAB Function2 : MATLAB Function  TreatAsAtomicUnit=on
  MATLAB Function5 : MATLAB Function  TreatAsAtomicUnit=on
  Memory1 : Memory  InitialCondition=1
  Memory{2..4,6..8} (6 alike) : Memory
  Memory5 : Memory  InitialCondition=[0 0 0]'
  Saturation : Saturate  UpperLimit=1  LowerLimit=-1
  Scope1 : Scope
  Scope7 : Scope  NumInputPorts=3
  Switch : Switch  Threshold=150  SaturateOnIntegerOverflow=off  InputSameDT=off
  To Workspace1 : ToWorkspace  VariableName=evsy1  SampleTime=-1
  To Workspace24 : ToWorkspace  VariableName=dist1  SampleTime=-1
  event_1 : MATLAB Function  TreatAsAtomicUnit=on
  event_x2 : MATLAB Function  TreatAsAtomicUnit=on
  memory_1 : MATLAB Function  TreatAsAtomicUnit=on
  U_ipos : Outport  VectorParamsAs1DForOutWhenUnconnected=off
  U_iyaw : Outport  Port=2  VectorParamsAs1DForOutWhenUnconnected=off
  tag scope: e_yaw1=global
  wires:
  state/1 -> Bus Selector1/1
  statej/1 -> Bus Selector2/1
  Bus Selector2/1 -> Demux1/1  "<xyz>"
  Demux4/1 -> memory_1/4(x), event_1/1(x), MATLAB Function/1(xi)
  Demux4/2 -> memory_1/5(y), event_1/2(y), MATLAB Function/2(yi)
  Demux1/1 -> MATLAB Function/4(xj)
  Demux1/2 -> MATLAB Function/5(yj)
  Discrete-Time Integrator1/1 -> MATLAB Function1/3(phiAlpha_int)
  MATLAB Function2/1(ui_gamma) -> Scope1/1, Memory5/1, MATLAB Function1/4(ui_gamma)
  statek/1 -> Bus Selector3/1
  Demux3/1 -> MATLAB Function/7(xk)
  Demux3/2 -> MATLAB Function/8(yk)
  Bus Selector3/1 -> Demux3/1  "<xyz>"
  MATLAB Function/1(phiAlpha) -> Gain2/1
  Demux4/3 -> memory_1/6(z), event_1/3(z), MATLAB Function/3(zi)
  Demux3/3 -> MATLAB Function/9(zk)
  Demux1/3 -> MATLAB Function/6(zj)
  statel/1 -> Bus Selector4/1
  Demux7/1 -> MATLAB Function/10(xl)
  Demux7/2 -> MATLAB Function/11(yl)
  Demux7/3 -> MATLAB Function/12(zl)
  Bus Selector4/1 -> Demux7/1  "<xyz>"
  Bus Selector1/2 -> [YAW]  "<YAW>"
  [YAW] -> MATLAB Function1/5(yaw)
  MATLAB Function1/2(ui_yaw) -> U_iyaw/1
  MATLAB Function1/3(eyaw) -> Memory1/1, Discrete-Time Integrator3/1
  Discrete-Time Integrator3/1 -> MATLAB Function1/6(ieyaw)
  [K_alpha] -> MATLAB Function1/7(KP)
  [params] -> MATLAB Function/25(params)
  statem/1 -> Bus Selector5/1
  Bus Selector5/1 -> Demux2/1  "<xyz>"
  Demux2/1 -> MATLAB Function/13(xm)
  Demux2/2 -> MATLAB Function/14(ym)
  Demux2/3 -> MATLAB Function/15(zm)
  Memory1/1 -> [e_yaw1]
  [e_yaw2] -> MATLAB Function1/8(eyaw2)
  [e_yaw3] -> MATLAB Function1/9(eyaw3)
  [e_yaw4] -> MATLAB Function1/10(eyaw4)
  [e_yaw5] -> MATLAB Function1/11(eyaw5)
  Discrete-Time Integrator4/1 -> MATLAB Function5/3(q_hat)
  Discrete-Time Integrator5/1 -> Saturation/1, MATLAB Function5/4(eta1)
  [L_obs] -> MATLAB Function5/1(L)
  MATLAB Function5/1(dot_hat_q) -> Discrete-Time Integrator4/1
  MATLAB Function1/1(Ui_pos) -> MATLAB Function5/6(u), U_ipos/1
  Bus Selector1/1 -> MATLAB Function5/2(q), Demux4/1  "<xyz>"
  MATLAB Function5/2(dot_eta) -> Discrete-Time Integrator5/1
  Discrete-Time Integrator6/1 -> MATLAB Function5/5(eta2)
  MATLAB Function5/3(ddot_eta) -> Discrete-Time Integrator6/1
  staten/1 -> Bus Selector6/1
  Demux6/1 -> MATLAB Function/16(xn)
  Demux6/2 -> MATLAB Function/17(yn)
  Demux6/3 -> MATLAB Function/18(zn)
  Bus Selector6/1 -> Demux6/1  "<xyz>"
  [e_yaw6] -> MATLAB Function1/12(eyaw6)
  stateo/1 -> Bus Selector7/1
  Demux8/1 -> MATLAB Function/19(xo)
  Demux8/2 -> MATLAB Function/20(yo)
  Demux8/3 -> MATLAB Function/21(zo)
  Bus Selector7/1 -> Demux8/1  "<xyz>"
  [e_yaw7] -> MATLAB Function1/13(eyaw7)
  statep/1 -> Bus Selector8/1
  Demux9/1 -> MATLAB Function/22(xp)
  Demux9/2 -> MATLAB Function/23(yp)
  Demux9/3 -> MATLAB Function/24(zp)
  Bus Selector8/1 -> Demux9/1  "<xyz>"
  [e_yaw8] -> MATLAB Function1/14(eyaw8)
  Demux5/1 -> MATLAB Function2/5(xr1)
  ref/1 -> Bus Selector/1
  Demux10/1 -> MATLAB Function2/8(xr2)
  [K_con] -> MATLAB Function2/18(K_cts)
  Discrete-Time Integrator2/1 -> MATLAB Function2/14(iep)
  ref1/1 -> Bus Selector9/1
  Demux10/3 -> MATLAB Function2/10(zr2)
  Demux10/2 -> MATLAB Function2/9(yr2)
  MATLAB Function2/2(ep) -> Discrete-Time Integrator2/1
  Bus Selector/1 -> Demux5/1  "<xi_d>"
  Demux5/3 -> MATLAB Function2/7(zr1)
  Bus Selector9/1 -> Demux10/1  "<xyz>"
  Demux5/2 -> MATLAB Function2/6(yr1)
  Saturation/1 -> To Workspace24/1, Gain1/1, Gain/1
  Switch/1 -> MATLAB Function1/1(eta)
  Gain/1 -> Switch/1
  [gaz_time] -> Switch/2
  Gain1/1 -> Switch/3
  Bus Selector10/1 -> Demux11/1  "<xyz>"
  Demux11/2 -> MATLAB Function2/12(yr3)
  Demux11/3 -> MATLAB Function2/13(zr3)
  ref2/1 -> Bus Selector10/1
  Demux11/1 -> MATLAB Function2/11(xr3)
  Memory2/1 -> memory_1/7("mx "), event_1/4(mx), [x_sam]
  event_1/1(norm_ex) -> [norm_ex], memory_1/1(ex)
  memory_1/1(mx) -> Memory2/1
  memory_1/2(my) -> Memory3/1
  memory_1/3(mz) -> Memory4/1
  Memory3/1 -> [y_sam], memory_1/8("my "), event_1/5(my)
  Memory4/1 -> memory_1/9("mz "), event_1/6(mz), [z_sam]
  event_1/2(norm_ey) -> [norm_ey], memory_1/2(ey)
  event_1/3(norm_ez) -> [norm_ez], memory_1/3(ez)
  [C0] -> event_1/7(c0)
  [x_sam] -> MATLAB Function2/2(xi)
  [y_sam] -> MATLAB Function2/3(yi)
  [z_sam] -> MATLAB Function2/4(zi)
  Memory5/1 -> MATLAB Function2/1(ui_prev)
  [norm_ex] -> MATLAB Function2/15(norm_ex)
  [norm_ey] -> MATLAB Function2/16(norm_ey)
  [norm_ez] -> MATLAB Function2/17(norm_ez)
  Gain2/1 -> MATLAB Function1/2(phiAlpha), Discrete-Time Integrator1/1
  Memory8/1 -> To Workspace1/1, event_x2/5("i2 ")
  event_x2/2(e_2) -> Scope7/2
  Memory7/1 -> event_x2/6("i3 ")
  event_x2/3(e_3) -> Scope7/3
  Memory6/1 -> event_x2/4("i1 ")
  event_x2/5(i2) -> Memory8/1
  event_x2/6(i3) -> Memory7/1
  [norm_ez] -> event_x2/3(e3)
  [norm_ey] -> event_x2/2(e2)
  event_x2/4(i1) -> Memory6/1
  [norm_ex] -> event_x2/1(e1)
  event_x2/1(e_1) -> Scope7/1
